simulink model "pmsgWindTurbineWithMpptBoostConverter"  (R2024b)
settings: Solver=ode23t  StartTime=0.0  StopTime=10  RelTol=1e-3
libraries: spsMeanLib x5, spsSeriesRLCBranchLib x4, spsCurrentMeasurementLib x3, spsVoltageMeasurementLib x3, spsRMSLib x2, spsDiodeLib x1, spsMosfetLib x1, spsPWMGeneratorDCDCLib x1, spsPermanentMagnetSynchronousMachineLib x1, spsWindTurbineLib x1, rllib x1, spsStairGeneratorLib x1
settings Model: Creator=Shashank  LastModifiedBy=ANANTHA KRISHNA S K

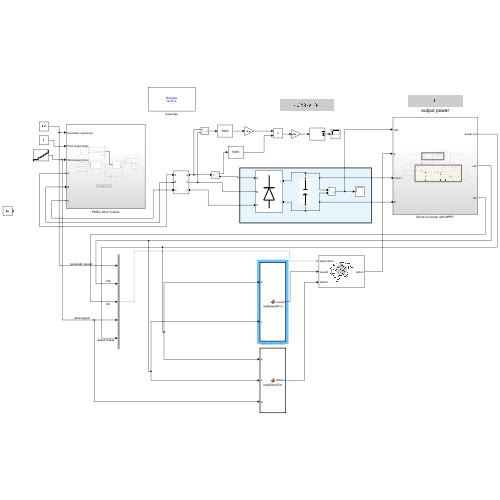
[thumbnail: Simulink's stored preview of the top-level diagram]
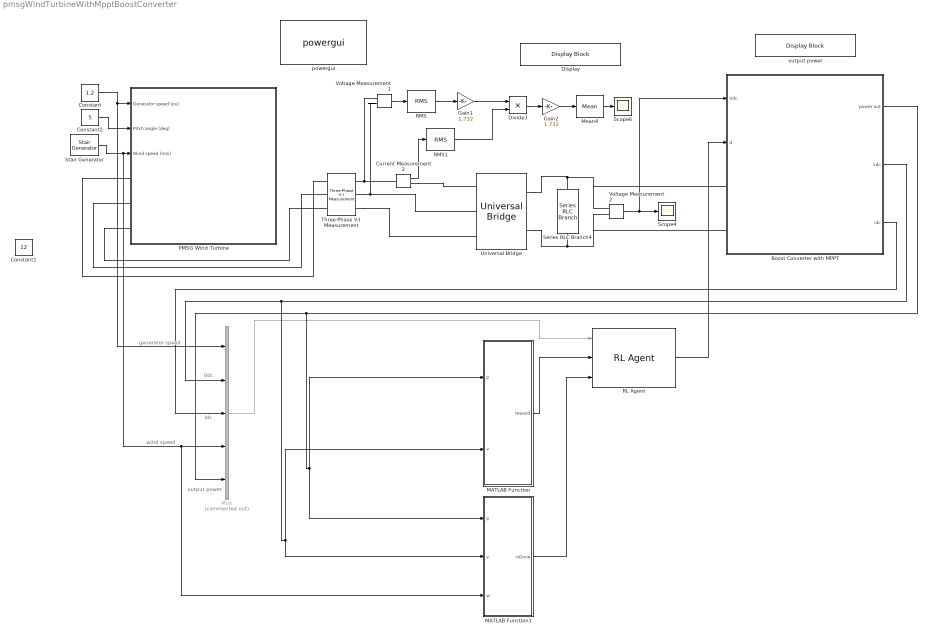
== system pmsgWindTurbineWithMpptBoostConverter ==
  note: output power
  note: Idc
  note: Vdc
  note: wind speed
  note: generator speed
  Boost Converter with MPPT : Subsystem
  Constant : Constant  Value=1.2
  Constant1 : Constant  Value=12
  Constant2 : Constant  Value=5
  Current Measurement2 : spsCurrentMeasurementLib/Current Measurement  PhasorSimulation=off  OutputType=Complex  PSBequivalent=0
  Display : DisplayBlock  LabelPosition=Hide  Transparency=1
  Divide3 : Product  Inputs=**
  Gain1 : Gain  Gain=1.732
  Gain2 : Gain  Gain=1.732
  MATLAB Function : MATLAB Function  TreatAsAtomicUnit=on
  MATLAB Function1 : MATLAB Function  TreatAsAtomicUnit=on
  Mean4 : spsMeanLib/Mean  Freq=50  Vinit=0  Ts=50e-6
  Mux : Mux  Commented=on  Inputs=5
  PMSG Wind Turbine : Subsystem
  RL Agent : rllib/RL Agent  Agent=agentObj  ExternalActionAsInput=off  ProvideLastAction=off  ProvideCumRwd=off  TreatAsDirectFeedthrough=on  UseStrictObservationDataTypes=off
  RMS : spsRMSLib/RMS  TrueRMS=on  Freq=50  RMSInit=120  Ts=50e-6
  RMS1 : spsRMSLib/RMS  TrueRMS=on  Freq=50  RMSInit=120  Ts=50e-6
  Scope4 : Scope
  Scope6 : Scope
  Series RLC Branch4 : spsSeriesRLCBranchLib/Series RLC Branch  LConnTagsString=__new0  RConnTagsString=__new0  BranchType=C  Resistance=1  Inductance=1e-3  SetiL0=off  InitialCurrent=0  Capacitance=11000e-6  Setx0=off  InitialVoltage=0  Measurements=None
  Stair Generator : spsStairGeneratorLib/Stair Generator  t=[0, 1, 3, 4, 5, 6, 7]  e=[5, 6, 7 ,8, 9, 10,12]  Ts=20e-6
  Three-Phase V-I Measurement : spsThreePhaseVIMeasurementLib/Three-Phase V-I Measurement  VoltageMeasurement=no  SetLabelV=off  LabelV=Vabc  Vpu=off  VpuLL=off  CurrentMeasurement=no  SetLabelI=off  LabelI=Iabc  Ipu=off  Pbase=100e6  Vbase=500e3  OutputType=Complex  PhasorSimulation=off  PSBequivalent=0
  Universal Bridge : spsUniversalBridgeLib/Universal Bridge  Arms=3  SnubberResistance=1e5  SnubberCapacitance=inf  Device=Diodes  Ron=1e-3  Lon=0  ForwardVoltages="[  0  0  ]"  ForwardVoltage=0  GTOparameters=[ 10e-6 , 20e-6 ]  IGBTparameters=[ 1e-6 , 2e-6 ]  Measurements=None  Measurements_2=None  converterType=Rectifier
  Voltage Measurement1 : spsVoltageMeasurementLib/Voltage Measurement  PhasorSimulation=off  OutputType=Complex  PSBequivalent=0
  Voltage Measurement2 : spsVoltageMeasurementLib/Voltage Measurement  PhasorSimulation=off  OutputType=Complex  PSBequivalent=0
  output power : DisplayBlock  LabelPosition=Hide  Transparency=1
  powergui : sps_lib/powergui  Priority=1  SimulationMode=Discrete  SampleTime=10e-6  frequency=60  Iterations=50  frequencyindice=0  Pbase=100e6  ErrMax=1e-4  UnitsV=kV  UnitsW=MW  buscounter=0  FunctionMessages=off  echomessages=off  EnableUseOfTLC=off  CurrentSourceSwitches=off  DisableSnubberDevices=off  DisableRonSwitches=off  DisableVfSwitches=off  DisplayEquations=off  AutomaticDiscreteSolvers=off  SolverType=Tustin/Backward Euler (TBE)  Interpol=off  ExternalGateDelay=off  methode=off  Ts=100  x0status=blocks  SPID=on  SwTol=0  HookPort=off  NonlinearTolerance=1e-4  nMaxIteration=100  ContinueOnMaxIteration=off  RestoreLinks=warning  ResistiveCurrentMeasurement=off  Frange=[0:2:500]  Ylog=off  Xlog=on  ShowGrid=off  save=off  variable=ZData  structure=0  ZoomFFT=off  StartTime=0.0  cycles=1  DisplayStyle=1  fundamental=60  FreqAxis=off  MaxFrequency=1000  frequencyindicesteady=1  RmsSteady=1  display=off
  wires:
  Voltage Measurement2/1 -> Boost Converter with MPPT/1(Vdc), Scope4/1
  Voltage Measurement1/1 -> RMS/1
  RMS/1 -> Gain1/1
  Gain1/1 -> Divide3/1
  RMS1/1 -> Divide3/2
  Divide3/1 -> Gain2/1
  Current Measurement2/1 -> RMS1/1
  Mean4/1 -> Scope6/1
  Gain2/1 -> Mean4/1
  Constant/1 -> Mux/1, PMSG Wind Turbine/1(Generator speed (pu))
  Constant2/1 -> PMSG Wind Turbine/2(Pitch angle (deg))
  Stair Generator/1 -> MATLAB Function1/3(w), Mux/4, PMSG Wind Turbine/3(Wind speed (m/s))
  Mux/1 -> RL Agent/1
  RL Agent/1 -> Boost Converter with MPPT/2(d)
  Boost Converter with MPPT/1(power out) -> MATLAB Function1/1(p), MATLAB Function/1(p), Mux/5
  Boost Converter with MPPT/2(vdc) -> MATLAB Function/2(v), MATLAB Function1/2(v), Mux/2
  Boost Converter with MPPT/3(idc) -> Mux/3
  MATLAB Function/1(reward) -> RL Agent/2
  MATLAB Function1/1(isDone) -> RL Agent/3
  connections:
  Universal Bridge/RConn1 -- Voltage Measurement2/LConn1 -- Boost Converter with MPPT/LConn1 -- Series RLC Branch4/LConn1
  Three-Phase V-I Measurement/RConn1 -- Current Measurement2/LConn1 -- Voltage Measurement1/LConn1
  Three-Phase V-I Measurement/RConn2 -- Voltage Measurement1/LConn2 -- Universal Bridge/LConn2
  Three-Phase V-I Measurement/RConn3 -- Universal Bridge/LConn3
  Current Measurement2/RConn1 -- Universal Bridge/LConn1
  PMSG Wind Turbine/LConn1 -- Three-Phase V-I Measurement/LConn1
  PMSG Wind Turbine/LConn2 -- Three-Phase V-I Measurement/LConn2
  PMSG Wind Turbine/LConn3 -- Three-Phase V-I Measurement/LConn3
  Universal Bridge/RConn2 -- Voltage Measurement2/LConn2 -- Boost Converter with MPPT/LConn2 -- Series RLC Branch4/RConn1

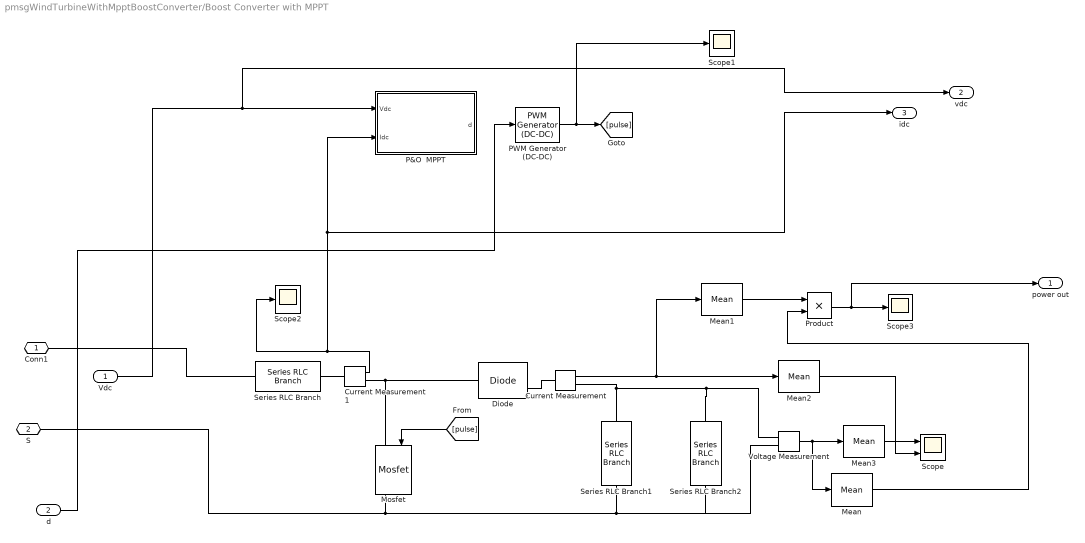
== system pmsgWindTurbineWithMpptBoostConverter/Boost Converter with MPPT ==
  Vdc : Inport
  d : Inport  Port=2
  Current Measurement : spsCurrentMeasurementLib/Current Measurement  PhasorSimulation=off  OutputType=Complex  PSBequivalent=0
  Current Measurement1 : spsCurrentMeasurementLib/Current Measurement  PhasorSimulation=off  OutputType=Complex  PSBequivalent=0
  Diode : spsDiodeLib/Diode  Ron=0.001  Lon=0  Vf=0.8  IC=0  UseSnubber=0  Rs=500  Cs=250e-9  Measurements=on
  Mean{,1..3} (4 alike) : spsMeanLib/Mean  Freq=50  Vinit=0  Ts=50e-6
  Mosfet : spsMosfetLib/Mosfet  Ron=0.1  Lon=0  Rd=0.01  Vfd=0  IC=0  Rs=1e5  Cs=inf  Measurements=on
  P&O  MPPT : Subsystem
  PWM Generator (DC-DC) : spsPWMGeneratorDCDCLib/PWM Generator (DC-DC)  Fsw=20000  Ts=0
  Product : Product
  Scope : Scope  NumInputPorts=2
  Scope1 : Scope
  Scope2 : Scope
  Scope3 : Scope
  Series RLC Branch : spsSeriesRLCBranchLib/Series RLC Branch  LConnTagsString=__new0  RConnTagsString=__new0  BranchType=L  Resistance=1  Inductance=250e-6  SetiL0=off  InitialCurrent=0  Capacitance=1e-6  Setx0=off  InitialVoltage=0  Measurements=None
  Series RLC Branch1 : spsSeriesRLCBranchLib/Series RLC Branch  LConnTagsString=__new0  RConnTagsString=__new0  BranchType=C  Resistance=1  Inductance=1e-3  SetiL0=off  InitialCurrent=0  Capacitance=270e-6  Setx0=off  InitialVoltage=0  Measurements=None
  Series RLC Branch2 : spsSeriesRLCBranchLib/Series RLC Branch  LConnTagsString=__new0  RConnTagsString=__new0  BranchType=R  Resistance=5.2  Inductance=1e-3  SetiL0=off  InitialCurrent=0  Capacitance=1e-6  Setx0=off  InitialVoltage=0  Measurements=None
  Voltage Measurement : spsVoltageMeasurementLib/Voltage Measurement  PhasorSimulation=off  OutputType=Complex  PSBequivalent=0
  Conn1 : PMIOPort  Side=Left
  S : PMIOPort  Port=2  Side=Left
  power out : Outport
  vdc : Outport  Port=2
  idc : Outport  Port=3
  wires:
  Product/1 -> power out/1, Scope3/1
  Vdc/1 -> vdc/1, P&O  MPPT/1(Vdc)
  [pulse] -> Mosfet/1
  Current Measurement1/1 -> idc/1, P&O  MPPT/2(Idc), Scope2/1
  Current Measurement/1 -> Mean1/1, Mean2/1
  Mean/1 -> Product/2
  Voltage Measurement/1 -> Mean/1, Mean3/1
  PWM Generator (DC-DC)/1 -> Scope1/1, [pulse]
  Mean3/1 -> Scope/1
  Mean2/1 -> Scope/2
  Mean1/1 -> Product/1
  d/1 -> PWM Generator (DC-DC)/1
  connections:
  Series RLC Branch2/LConn1 -- Voltage Measurement/LConn1 -- Current Measurement/RConn1 -- Series RLC Branch1/LConn1
  Diode/LConn1 -- Current Measurement1/RConn1 -- Mosfet/LConn1
  Current Measurement/LConn1 -- Diode/RConn1
  Current Measurement1/LConn1 -- Series RLC Branch/RConn1
  Series RLC Branch1/RConn1 -- Series RLC Branch2/RConn1 -- Voltage Measurement/LConn2 -- Mosfet/RConn1 -- S/RConn1
  Series RLC Branch/LConn1 -- Conn1/RConn1

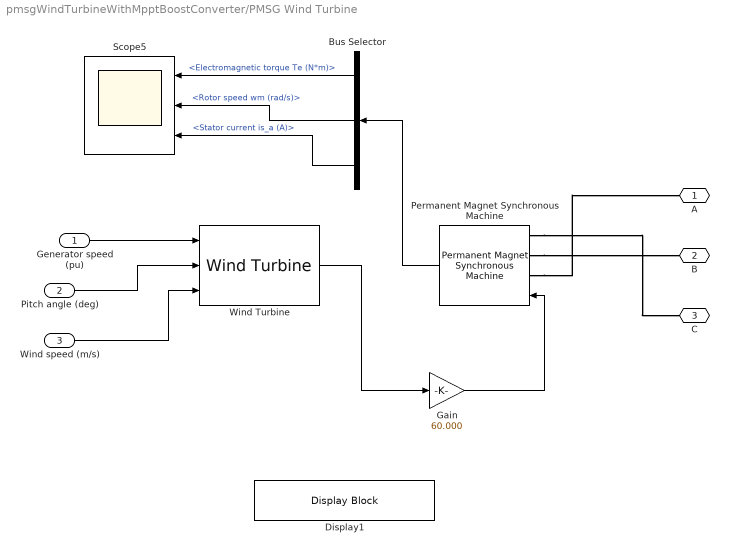
== system pmsgWindTurbineWithMpptBoostConverter/PMSG Wind Turbine ==
  Generator speed (pu) : Inport
  Pitch angle (deg) : Inport  Port=2
  Wind speed (m/s) : Inport  Port=3
  Bus Selector : BusSelector  OutputSignals=Electromagnetic torque Te (N*m),Rotor speed wm (rad/s),Stator current is_a (A)
  Display1 : DisplayBlock  LabelPosition=Hide  Transparency=1
  Gain : Gain  Gain=60.000
  Permanent Magnet Synchronous Machine : spsPermanentMagnetSynchronousMachineLib/Permanent Magnet Synchronous Machine  NbPhases=3  FluxDistribution=Sinusoidal  RotorType=Salient-pole  MechanicalLoad=Torque Tm  PresetModel="14:  67.27 Nm 560 Vdc 1700 RPM - 70.2 Nm"  ShowDetailedParameters=on  MeasurementBus=off  Resistance=0.085  Inductance=8.5e-3  dqInductances=[0.0009025 0.0009975]  La=0.000395  MachineConstant=Flux linkage established by magnets (V.s)  Flux=0.192  VoltageCst=139.2998  TorqueCst=1.152  Flat=120  Mechanical=[0.008 0.001147 4 0]  PolePairs=4  InitialConditions=[0,0, 0,0]  InitialConditions5ph=[0 0 0 0 0 0]  RefAngle=90 degrees behind phase A axis (modified Park)  IterativeDiscreteModel=Trapezoidal non iterative  TsBlock=-1  TsPowergui=0
  Scope5 : Scope  NumInputPorts=3
  Wind Turbine : spsWindTurbineLib/Wind Turbine  Pnom=1e3  Pelec_base=1e3/0.9  wind_base=12  P_wind_base=0.85  speed_nom=1.2  pitch_angle=0  c1_c6="[0.51763          116          0.4            5           21     0.006795]"  cp_nom=0.48  lambda_nom=8.1
  A : PMIOPort  Side=Left
  B : PMIOPort  Port=2  Side=Left
  C : PMIOPort  Port=3  Side=Left
  wires:
  Permanent Magnet Synchronous Machine/1 -> Bus Selector/1
  Bus Selector/2 -> Scope5/2  "<Rotor speed wm (rad/s)>"
  Bus Selector/1 -> Scope5/1  "<Electromagnetic torque Te (N*m)>"
  Generator speed (pu)/1 -> Wind Turbine/1
  Bus Selector/3 -> Scope5/3  "<Stator current is_a (A)>"
  Wind Turbine/1 -> Gain/1
  Gain/1 -> Permanent Magnet Synchronous Machine/1
  Wind speed (m/s)/1 -> Wind Turbine/3
  Pitch angle (deg)/1 -> Wind Turbine/2
  connections:
  Permanent Magnet Synchronous Machine/LConn3 -- C/RConn1
  Permanent Magnet Synchronous Machine/LConn1 -- A/RConn1
  Permanent Magnet Synchronous Machine/LConn2 -- B/RConn1

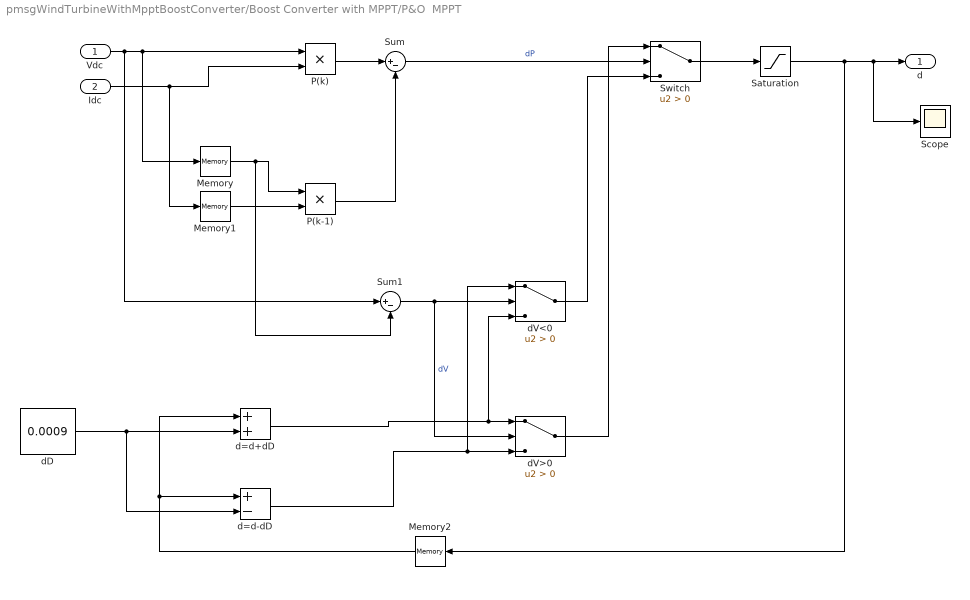
== system pmsgWindTurbineWithMpptBoostConverter/Boost Converter with MPPT/P&O  MPPT ==
  Vdc : Inport
  Idc : Inport  Port=2
  Memory : Memory  InheritSampleTime=on  LinearizeAsDelay=on
  Memory1 : Memory  InheritSampleTime=on  LinearizeAsDelay=on
  Memory2 : Memory
  P(k) : Product
  P(k-1) : Product
  Saturation : Saturate  UpperLimit=0.6  LowerLimit=0.2
  Scope : Scope
  Sum : Sum  Inputs=|+-
  Sum1 : Sum  Inputs=|+-
  Switch : Switch  Criteria=u2 > Threshold  SaturateOnIntegerOverflow=off  InputSameDT=off
  d=d+dD : Sum
  d=d-dD : Sum  Inputs=+-
  dD : Constant  Value=0.0009
  dV<0 : Switch  Criteria=u2 > Threshold  SaturateOnIntegerOverflow=off  InputSameDT=off
  dV>0 : Switch  Criteria=u2 > Threshold  SaturateOnIntegerOverflow=off  InputSameDT=off
  d : Outport
  wires:
  Memory/1 -> Sum1/2, P(k-1)/1
  Memory1/1 -> P(k-1)/2
  P(k)/1 -> Sum/1
  P(k-1)/1 -> Sum/2
  Sum/1 -> Switch/2  "dP"
  Sum1/1 -> dV>0/2, dV<0/2  "dV"
  Memory2/1 -> d=d-dD/1, d=d+dD/1
  dD/1 -> d=d-dD/2, d=d+dD/2
  d=d+dD/1 -> dV<0/3, dV>0/1
  d=d-dD/1 -> dV<0/1, dV>0/3
  dV>0/1 -> Switch/1
  dV<0/1 -> Switch/3
  Switch/1 -> Saturation/1
  Saturation/1 -> Memory2/1, Scope/1, d/1
  Vdc/1 -> Sum1/1, Memory/1, P(k)/1
  Idc/1 -> Memory1/1, P(k)/2

== matlab function pmsgWindTurbineWithMpptBoostConverter/MATLAB Function1 ==
  data: p input; v input; isDone output; w input
function isDone = myIsDoneFcn(p,v,w)
    Vdc = v;   
    Pout = p;  
    WindSpeed = w; 
    
    % Safety limits
    if (Vdc > 450 || Pout < 100 || WindSpeed > 25) 
        isDone = true; 
    else
        isDone = false; 
    end
    
end

== matlab function pmsgWindTurbineWithMpptBoostConverter/MATLAB Function ==
  data: p input; v input; reward output
function reward = myRewardFcn(p, v)
    Pout = p;   
    Vdc = v;   
    Vref = 400;     
    lambda = 0.1;   
    
    reward = Pout - lambda * abs(Vdc - Vref);
    disp(['Reward: ', sprintf('%f', reward)
])

end
